simulink model "Task5_sim"  (R2014a)
settings: Solver=ode45  StartTime=3  StopTime=5  RelTol=1e-3
settings Model: Creator=bunka  LastModifiedBy=bunka

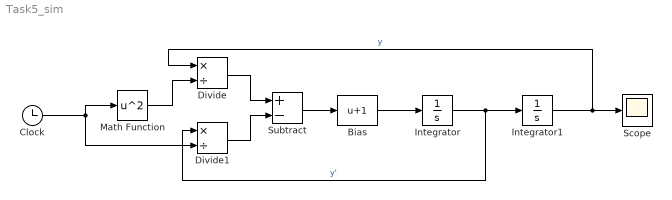
== system Task5_sim ==
  Bias : Bias  Bias=1
  Clock : Clock
  Divide : Product  Inputs=*/
  Divide1 : Product  Inputs=*/
  Integrator : Integrator  InitialCondition=3
  Integrator1 : Integrator  InitialCondition=6
  Math Function : Math  Operator=square  SaturateOnIntegerOverflow=on
  Scope : Scope
  Subtract : Sum  Inputs=+-
  wires:
  Integrator1/1 -> Divide/1, Scope/1  "y"
  Integrator/1 -> Divide1/1, Integrator1/1  "y'"
  Bias/1 -> Integrator/1
  Subtract/1 -> Bias/1
  Divide1/1 -> Subtract/2
  Divide/1 -> Subtract/1
  Clock/1 -> Divide1/2, Math Function/1
  Math Function/1 -> Divide/2
